simulink model "controlGPI_pos_6dof_sinMI"  (R2023b)
settings: Solver=ode45  StartTime=0.0  StopTime=tsim  FixedStep=tstep  MaxStep=tstep  RelTol=tstep/10
undefined symbols (not defined in the file): contr_robot_params, ddq, dq, ndof, NN_Bspline_params, NN_RBF_params, nn_select, Pc, q0, q_cero, q_eq, robot_params, t_qeq_init, t_tr_init, t_trtr, tau_L, tau_L_mags, tr_muestra, tr_ref, Wc, Zc
libraries: simulink x2
(part 1 of 2)
settings Model: Creator=HP  LastModifiedBy=HP

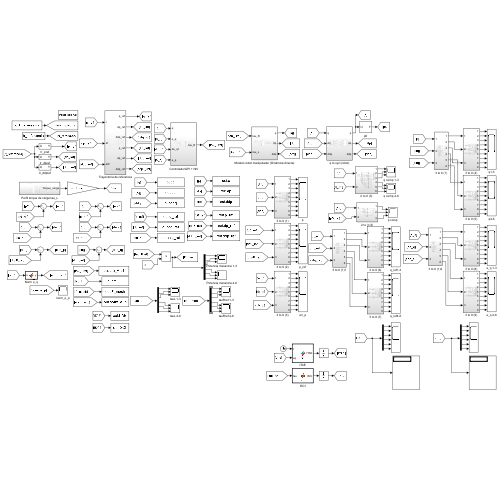
[thumbnail: Simulink's stored preview of the top-level diagram]
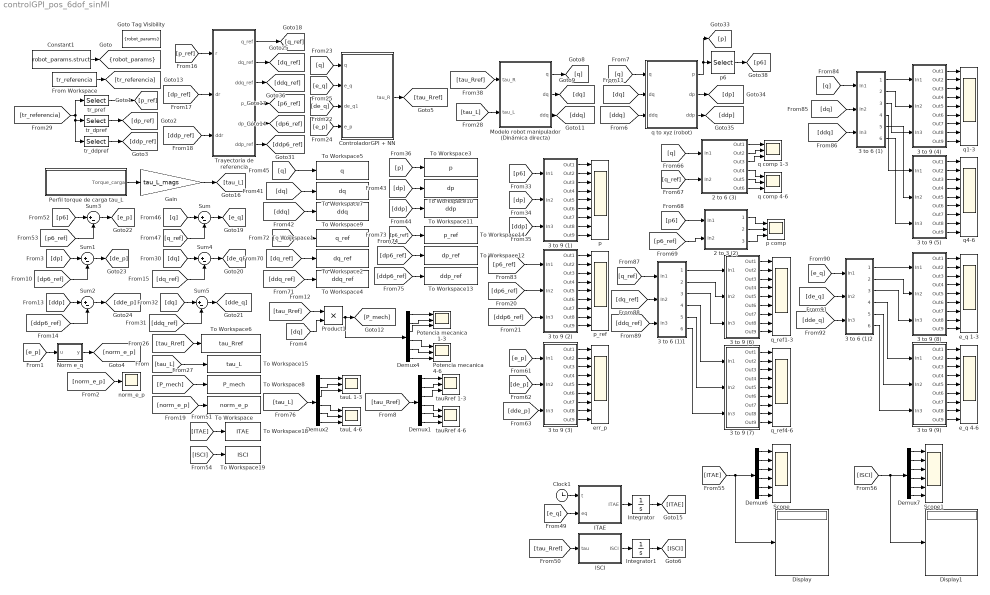
== system controlGPI_pos_6dof_sinMI ==
  2 to 3 (2) : Subsystem
  2 to 6 (3) : Subsystem
  3 to 6 (1) : Subsystem
  3 to 6 (1)1 : Subsystem
  3 to 6 (1)2 : Subsystem
  3 to 9 (1) : Subsystem
  3 to 9 (2) : Subsystem
  3 to 9 (3) : Subsystem
  3 to 9 (4) : Subsystem
  3 to 9 (5) : Subsystem
  3 to 9 (6) : Subsystem
  3 to 9 (7) : Subsystem
  3 to 9 (8) : Subsystem
  3 to 9 (9) : Subsystem
  Clock1 : Clock
  Constant1 : Constant  Value=robot_params.struct  OutDataTypeStr=Bus: robot_params_bus
  ControladorGPI + NN : Subsystem
  Demux{1..2,4,6..7} (5 alike) : Demux  Outputs=6
  Display : Display
  Display1 : Display
  From Workspace : FromWorkspace  VariableName=tr_referencia
  Gain : Gain  Gain=tau_L_mags
  Goto Tag Visibility : GotoTagVisibility  GotoTag=robot_params
  ISCI : MATLAB Function  TreatAsAtomicUnit=on
  ITAE : MATLAB Function  TreatAsAtomicUnit=on
  Integrator : Integrator
  Integrator1 : Integrator
  Modelo robot manipulador (Dinámica directa) : Subsystem
  Norm e_q : MATLAB Function  TreatAsAtomicUnit=on
  Perfil torque de carga tau_L : Subsystem
  Potencia mecanica 1-3 : Scope  NumInputPorts=3
  Potencia mecanica 4-6 : Scope  NumInputPorts=3
  Product1 : Product
  Scope : Scope  NumInputPorts=6
  Scope1 : Scope  NumInputPorts=6
  Sum{,1..5} (6 alike) : Sum  Inputs=|+-
  To Workspace : ToWorkspace  VariableName=norm_e_p  SaveFormat=Timeseries  SampleTime=-1
  To Workspace1 : ToWorkspace  VariableName=q_ref  SaveFormat=Timeseries  SampleTime=-1
  To Workspace10 : ToWorkspace  VariableName=dp  SaveFormat=Timeseries  SampleTime=-1
  To Workspace11 : ToWorkspace  VariableName=ddp  SaveFormat=Timeseries  SampleTime=-1
  To Workspace12 : ToWorkspace  VariableName=dp_ref  SaveFormat=Timeseries  SampleTime=-1
  To Workspace13 : ToWorkspace  VariableName=ddp_ref  SaveFormat=Timeseries  SampleTime=-1
  To Workspace14 : ToWorkspace  VariableName=p_ref  SaveFormat=Timeseries  SampleTime=-1
  To Workspace15 : ToWorkspace  VariableName=tau_L  SaveFormat=Timeseries  SampleTime=-1
  To Workspace18 : ToWorkspace  VariableName=ITAE  SampleTime=-1
      settings: MaxDataPoints=1
  To Workspace19 : ToWorkspace  VariableName=ISCI  SampleTime=-1
      settings: MaxDataPoints=1
  To Workspace2 : ToWorkspace  VariableName=dq_ref  SaveFormat=Timeseries  SampleTime=-1
  To Workspace3 : ToWorkspace  VariableName=p  SaveFormat=Timeseries  SampleTime=-1
  To Workspace4 : ToWorkspace  VariableName=ddq_ref  SaveFormat=Timeseries  SampleTime=-1
  To Workspace5 : ToWorkspace  VariableName=q  SaveFormat=Timeseries  SampleTime=-1
  To Workspace6 : ToWorkspace  VariableName=tau_Rref  SaveFormat=Timeseries  SampleTime=-1
  To Workspace7 : ToWorkspace  VariableName=dq  SaveFormat=Timeseries  SampleTime=-1
  To Workspace8 : ToWorkspace  VariableName=P_mech  SaveFormat=Timeseries  SampleTime=-1
  To Workspace9 : ToWorkspace  VariableName=ddq  SaveFormat=Timeseries  SampleTime=-1
  Trayectoria de referencia : Subsystem
  e_q 1-3 : Scope  NumInputPorts=9
  e_q 4-6 : Scope  NumInputPorts=9
  err_p : Scope  NumInputPorts=9
  norm_e_p : Scope
  p : Scope  NumInputPorts=9
  p comp : Scope  NumInputPorts=3
  p6 : Selector  NumberOfDimensions=2  InputPortWidth=3  IndexOptions=Index vector (dialog),Index vector (dialog)  Indices=[1:3],6  OutputSizes=1,1
  p_ref : Scope  NumInputPorts=9
  q comp 1-3 : Scope  NumInputPorts=3
  q comp 4-6 : Scope  NumInputPorts=3
  q to xyz (robot) : Subsystem
  q1-3 : Scope  NumInputPorts=9
  q4-6 : Scope  NumInputPorts=9
  q_ref1-3 : Scope  NumInputPorts=9
  q_ref4-6 : Scope  NumInputPorts=9
  tauL 1-3 : Scope  NumInputPorts=3
  tauL 4-6 : Scope  NumInputPorts=3
  tauRref 1-3 : Scope  NumInputPorts=3
  tauRref 4-6 : Scope  NumInputPorts=3
  tr_ddpref : Selector  NumberOfDimensions=2  InputPortWidth=3  IndexOptions=Index vector (dialog),Index vector (dialog)  Indices=[7:9],1  OutputSizes=1,1
  tr_dpref : Selector  NumberOfDimensions=2  InputPortWidth=3  IndexOptions=Index vector (dialog),Index vector (dialog)  Indices=[4:6],1  OutputSizes=1,1
  tr_pref : Selector  NumberOfDimensions=2  InputPortWidth=3  IndexOptions=Index vector (dialog),Index vector (dialog)  Indices=[1:3],1  OutputSizes=1,1
  tag scope: robot_params=scoped
  wires:
  [ddp] -> To Workspace11/1
  [P_mech] -> To Workspace8/1
  [dq] -> To Workspace7/1
  [q] -> To Workspace5/1
  [tau_Rref] -> To Workspace6/1
  [dp] -> To Workspace10/1
  [p] -> To Workspace3/1
  [ddq] -> To Workspace9/1
  [dq_ref] -> To Workspace2/1
  [ddq_ref] -> To Workspace4/1
  [q_ref] -> To Workspace1/1
  [p6_ref] -> To Workspace14/1
  [dp6_ref] -> To Workspace12/1
  [ddp6_ref] -> To Workspace13/1
  [tau_Rref] -> Modelo robot manipulador (Dinámica directa)/1(tau_R)
  [tau_L] -> Modelo robot manipulador (Dinámica directa)/2(tau_L)
  p6/1 -> [p6]
  q to xyz (robot)/1(p) -> p6/1, [p]
  [q] -> q to xyz (robot)/1(q)
  [dq] -> q to xyz (robot)/2(dq)
  [ddq] -> q to xyz (robot)/3(ddq)
  q to xyz (robot)/2(dp) -> [dp]
  q to xyz (robot)/3(ddp) -> [ddp]
  Modelo robot manipulador (Dinámica directa)/3(ddq) -> [ddq]
  Modelo robot manipulador (Dinámica directa)/2(dq) -> [dq]
  Modelo robot manipulador (Dinámica directa)/1(q) -> [q]
  2 to 6 (3)/6(Out6) -> q comp 4-6/3
  Demux4/2 -> Potencia mecanica 1-3/2
  2 to 6 (3)/5(Out5) -> q comp 4-6/2
  Demux1/4 -> tauRref 4-6/1
  2 to 6 (3)/3(Out3) -> q comp 1-3/3
  2 to 6 (3)/2(Out2) -> q comp 1-3/2
  3 to 9 (1)/4(Out4) -> p/4
  3 to 9 (2)/3(Out3) -> p_ref/3
  3 to 9 (3)/3(Out3) -> err_p/3
  3 to 9 (7)/9(Out9) -> q_ref4-6/9
  3 to 9 (4)/4(Out4) -> q1-3/4
  Demux2/5 -> tauL 4-6/2
  [tau_Rref] -> Demux1/1
  3 to 9 (1)/2(Out2) -> p/2
  [de_q] -> 3 to 6 (1)2/2(In2)
  Demux4/3 -> Potencia mecanica 1-3/3
  3 to 9 (3)/8(Out8) -> err_p/8
  2 to 3 (2)/3(3) -> p comp/3
  3 to 9 (5)/4(Out4) -> q4-6/4
  3 to 6 (1)/4(Out4) -> 3 to 9 (5)/1(In1)
  [dq] -> Product1/2
  3 to 6 (1)2/1(Out1) -> 3 to 9 (8)/1(In1)
  Demux2/3 -> tauL 1-3/3
  3 to 9 (6)/9(Out9) -> q_ref1-3/9
  3 to 9 (3)/4(Out4) -> err_p/4
  3 to 9 (7)/4(Out4) -> q_ref4-6/4
  3 to 9 (4)/1(Out1) -> q1-3/1
  3 to 9 (1)/9(Out9) -> p/9
  3 to 9 (2)/7(Out7) -> p_ref/7
  Product1/1 -> Demux4/1, [P_mech]
  Demux4/6 -> Potencia mecanica 4-6/3
  3 to 9 (1)/7(Out7) -> p/7
  3 to 9 (1)/6(Out6) -> p/6
  [dde_p] -> 3 to 9 (3)/3(In3)
  Demux4/4 -> Potencia mecanica 4-6/1
  3 to 9 (7)/1(Out1) -> q_ref4-6/1
  3 to 9 (4)/8(Out8) -> q1-3/8
  3 to 9 (4)/3(Out3) -> q1-3/3
  Demux2/1 -> tauL 1-3/1
  3 to 9 (2)/5(Out5) -> p_ref/5
  Demux1/1 -> tauRref 1-3/1
  3 to 9 (2)/9(Out9) -> p_ref/9
  3 to 6 (1)1/3(Out3) -> 3 to 9 (6)/3(In3)
  3 to 6 (1)/5(Out5) -> 3 to 9 (5)/2(In2)
  3 to 9 (5)/8(Out8) -> q4-6/8
  3 to 9 (4)/5(Out5) -> q1-3/5
  3 to 6 (1)1/1(Out1) -> 3 to 9 (6)/1(In1)
  3 to 9 (3)/2(Out2) -> err_p/2
  3 to 9 (8)/5(Out5) -> e_q 1-3/5
  3 to 9 (6)/1(Out1) -> q_ref1-3/1
  3 to 9 (2)/4(Out4) -> p_ref/4
  3 to 9 (5)/7(Out7) -> q4-6/7
  Demux2/4 -> tauL 4-6/1
  Demux2/2 -> tauL 1-3/2
  [ddp6_ref] -> 3 to 9 (2)/3(In3)
  Demux2/6 -> tauL 4-6/3
  3 to 6 (1)1/2(Out2) -> 3 to 9 (6)/2(In2)
  3 to 9 (7)/2(Out2) -> q_ref4-6/2
  3 to 9 (1)/1(Out1) -> p/1
  3 to 9 (3)/9(Out9) -> err_p/9
  3 to 9 (8)/1(Out1) -> e_q 1-3/1
  3 to 9 (3)/1(Out1) -> err_p/1
  3 to 9 (2)/6(Out6) -> p_ref/6
  Demux1/3 -> tauRref 1-3/3
  Demux1/5 -> tauRref 4-6/2
  3 to 9 (6)/4(Out4) -> q_ref1-3/4
  3 to 6 (1)1/5(Out5) -> 3 to 9 (7)/2(In2)
  Demux1/6 -> tauRref 4-6/3
  3 to 9 (8)/8(Out8) -> e_q 1-3/8
  3 to 9 (6)/3(Out3) -> q_ref1-3/3
  Demux1/2 -> tauRref 1-3/2
  3 to 6 (1)2/6(Out6) -> 3 to 9 (9)/3(In3)
  [tau_L] -> Demux2/1
  [dde_q] -> 3 to 6 (1)2/3(In3)
  3 to 9 (8)/2(Out2) -> e_q 1-3/2
  3 to 9 (8)/3(Out3) -> e_q 1-3/3
  3 to 9 (7)/3(Out3) -> q_ref4-6/3
  [de_p] -> 3 to 9 (3)/2(In2)
  [dp] -> 3 to 9 (1)/2(In2)
  3 to 9 (2)/8(Out8) -> p_ref/8
  3 to 6 (1)/1(Out1) -> 3 to 9 (4)/1(In1)
  3 to 9 (5)/3(Out3) -> q4-6/3
  [dq_ref] -> 3 to 6 (1)1/2(In2)
  3 to 9 (9)/8(Out8) -> e_q 4-6/8
  3 to 9 (6)/6(Out6) -> q_ref1-3/6
  3 to 9 (7)/8(Out8) -> q_ref4-6/8
  3 to 9 (8)/9(Out9) -> e_q 1-3/9
  [dp6_ref] -> 3 to 9 (2)/2(In2)
  3 to 9 (4)/6(Out6) -> q1-3/6
  3 to 9 (3)/6(Out6) -> err_p/6
  3 to 9 (6)/2(Out2) -> q_ref1-3/2
  3 to 9 (5)/6(Out6) -> q4-6/6
  3 to 6 (1)2/3(Out3) -> 3 to 9 (8)/3(In3)
  3 to 6 (1)1/4(Out4) -> 3 to 9 (7)/1(In1)
  3 to 9 (1)/8(Out8) -> p/8
  [tau_Rref] -> Product1/1
  3 to 9 (3)/7(Out7) -> err_p/7
  [q] -> 3 to 6 (1)/1(In1)
  2 to 3 (2)/1(1) -> p comp/1
  [ddq_ref] -> 3 to 6 (1)1/3(In3)
  3 to 9 (2)/2(Out2) -> p_ref/2
  3 to 9 (8)/4(Out4) -> e_q 1-3/4
  [dq] -> 3 to 6 (1)/2(In2)
  3 to 6 (1)2/2(Out2) -> 3 to 9 (8)/2(In2)
  3 to 9 (4)/7(Out7) -> q1-3/7
  [p6] -> 3 to 9 (1)/1(In1)
  3 to 6 (1)/6(Out6) -> 3 to 9 (5)/3(In3)
  3 to 9 (9)/5(Out5) -> e_q 4-6/5
  Demux4/5 -> Potencia mecanica 4-6/2
  3 to 9 (9)/4(Out4) -> e_q 4-6/4
  3 to 6 (1)2/4(Out4) -> 3 to 9 (9)/1(In1)
  3 to 9 (8)/6(Out6) -> e_q 1-3/6
  2 to 6 (3)/1(Out1) -> q comp 1-3/1
  [p6_ref] -> 3 to 9 (2)/1(In1)
  [e_p] -> 3 to 9 (3)/1(In1)
  2 to 6 (3)/4(Out4) -> q comp 4-6/1
  3 to 9 (1)/3(Out3) -> p/3
  3 to 6 (1)2/5(Out5) -> 3 to 9 (9)/2(In2)
  [p6] -> 2 to 3 (2)/1(In1)
  3 to 9 (4)/2(Out2) -> q1-3/2
  3 to 9 (9)/6(Out6) -> e_q 4-6/6
  [q] -> 2 to 6 (3)/1(In1)
  3 to 6 (1)/2(Out2) -> 3 to 9 (4)/2(In2)
  3 to 9 (3)/5(Out5) -> err_p/5
  3 to 9 (8)/7(Out7) -> e_q 1-3/7
  3 to 9 (5)/5(Out5) -> q4-6/5
  3 to 6 (1)1/6(Out6) -> 3 to 9 (7)/3(In3)
  3 to 9 (1)/5(Out5) -> p/5
  3 to 9 (2)/1(Out1) -> p_ref/1
  3 to 9 (7)/5(Out5) -> q_ref4-6/5
  3 to 9 (5)/9(Out9) -> q4-6/9
  3 to 9 (7)/6(Out6) -> q_ref4-6/6
  3 to 6 (1)/3(Out3) -> 3 to 9 (4)/3(In3)
  [q_ref] -> 2 to 6 (3)/2(In2)
  3 to 9 (9)/7(Out7) -> e_q 4-6/7
  2 to 3 (2)/2(2) -> p comp/2
  3 to 9 (7)/7(Out7) -> q_ref4-6/7
  3 to 9 (5)/1(Out1) -> q4-6/1
  3 to 9 (9)/3(Out3) -> e_q 4-6/3
  3 to 9 (4)/9(Out9) -> q1-3/9
  3 to 9 (6)/5(Out5) -> q_ref1-3/5
  Demux4/1 -> Potencia mecanica 1-3/1
  3 to 9 (6)/8(Out8) -> q_ref1-3/8
  3 to 9 (9)/2(Out2) -> e_q 4-6/2
  [ddp] -> 3 to 9 (1)/3(In3)
  [p6_ref] -> 2 to 3 (2)/2(In2)
  [e_q] -> 3 to 6 (1)2/1(In1)
  3 to 9 (9)/9(Out9) -> e_q 4-6/9
  3 to 9 (9)/1(Out1) -> e_q 4-6/1
  [q_ref] -> 3 to 6 (1)1/1(In1)
  3 to 9 (6)/7(Out7) -> q_ref1-3/7
  [ddq] -> 3 to 6 (1)/3(In3)
  3 to 9 (5)/2(Out2) -> q4-6/2
  tr_pref/1 -> [p_ref]
  tr_ddpref/1 -> [ddp_ref]
  [tr_referencia] -> tr_dpref/1, tr_ddpref/1, tr_pref/1
  Constant1/1 -> [robot_params]
  tr_dpref/1 -> [dp_ref]
  From Workspace/1 -> [tr_referencia]
  Trayectoria de referencia/4(p_ref) -> [p6_ref]
  Trayectoria de referencia/5(dp_ref) -> [dp6_ref]
  Trayectoria de referencia/3(ddq_ref) -> [ddq_ref]
  Trayectoria de referencia/2(dq_ref) -> [dq_ref]
  [p_ref] -> Trayectoria de referencia/1(r)
  [ddp_ref] -> Trayectoria de referencia/3(ddr)
  Trayectoria de referencia/6(ddp_ref) -> [ddp6_ref]
  Trayectoria de referencia/1(q_ref) -> [q_ref]
  [dp_ref] -> Trayectoria de referencia/2(dr)
  Sum1/1 -> [de_p]
  [norm_e_p] -> norm_e_p/1
  Sum2/1 -> [dde_p]
  Norm e_q/1(y) -> [norm_e_p]
  [p6] -> Sum3/1
  [q_ref] -> Sum/2
  Sum3/1 -> [e_p]
  Sum/1 -> [e_q]
  [e_p] -> Norm e_q/1(u)
  [q] -> Sum/1
  [p6_ref] -> Sum3/2
  [norm_e_p] -> To Workspace/1
  [e_q] -> ControladorGPI + NN/2(e_q)
  ControladorGPI + NN/1(tau_R) -> [tau_Rref]
  [de_q] -> ControladorGPI + NN/3(de_q1)
  [q] -> ControladorGPI + NN/1(q)
  [e_p] -> ControladorGPI + NN/4(e_p)
  [dp] -> Sum1/1
  [dp6_ref] -> Sum1/2
  [ddp] -> Sum2/1
  [ddp6_ref] -> Sum2/2
  [dq_ref] -> Sum4/2
  [dq] -> Sum4/1
  Sum4/1 -> [de_q]
  [ddq_ref] -> Sum5/2
  [dq] -> Sum5/1
  Sum5/1 -> [dde_q]
  Perfil torque de carga tau_L/1(Torque_carga) -> Gain/1
  Gain/1 -> [tau_L]
  [tau_L] -> To Workspace15/1
  Demux6/6 -> Scope/6
  Demux7/6 -> Scope1/6
  Demux7/5 -> Scope1/5
  ITAE/1(ITAE) -> Integrator/1
  [tau_Rref] -> ISCI/1(tau)
  Integrator/1 -> [ITAE]
  Integrator1/1 -> [ISCI]
  Demux6/5 -> Scope/5
  ISCI/1(ISCI) -> Integrator1/1
  [e_q] -> ITAE/2(eq)
  Clock1/1 -> ITAE/1(t)
  [ITAE] -> Display/1, Demux6/1
  [ISCI] -> Display1/1, Demux7/1
  Demux6/1 -> Scope/1
  Demux6/2 -> Scope/2
  Demux6/3 -> Scope/3
  Demux6/4 -> Scope/4
  Demux7/1 -> Scope1/1
  Demux7/2 -> Scope1/2
  Demux7/3 -> Scope1/3
  Demux7/4 -> Scope1/4
  [ITAE] -> To Workspace18/1
  [ISCI] -> To Workspace19/1

== system controlGPI_pos_6dof_sinMI/2 to 3 (2) ==
  In1 : Inport
  In2 : Inport  Port=2
  Demux3 : Demux  Outputs=3
  Demux4 : Demux  Outputs=3
  Mux10 : Mux  Inputs=2
  Mux8 : Mux  Inputs=2
  Mux9 : Mux  Inputs=2
  1 : Outport
  2 : Outport  Port=2
  3 : Outport  Port=3
  wires:
  Demux4/3 -> Mux10/2
  Demux3/1 -> Mux8/1
  Demux3/2 -> Mux9/1
  Mux9/1 -> 2/1
  Demux4/2 -> Mux9/2
  Demux4/1 -> Mux8/2
  Demux3/3 -> Mux10/1
  Mux8/1 -> 1/1
  Mux10/1 -> 3/1
  In1/1 -> Demux3/1
  In2/1 -> Demux4/1

== system controlGPI_pos_6dof_sinMI/2 to 6 (3) ==
  In1 : Inport
  In2 : Inport  Port=2
  Demux4 : Demux  Outputs=6
  Demux6 : Demux  Outputs=6
  Mux{,1..5} (6 alike) : Mux  Inputs=2
  Out1 : Outport
  Out2 : Outport  Port=2
  Out3 : Outport  Port=3
  Out4 : Outport  Port=4
  Out5 : Outport  Port=5
  Out6 : Outport  Port=6
  wires:
  In2/1 -> Demux6/1
  Demux4/3 -> Mux2/1
  Demux4/5 -> Mux4/1
  Demux4/6 -> Mux5/1
  Demux6/5 -> Mux4/2
  Demux4/1 -> Mux/1
  Demux6/6 -> Mux5/2
  In1/1 -> Demux4/1
  Demux4/4 -> Mux3/1
  Demux6/2 -> Mux1/2
  Demux6/4 -> Mux3/2
  Demux6/1 -> Mux/2
  Demux4/2 -> Mux1/1
  Demux6/3 -> Mux2/2
  Mux/1 -> Out1/1
  Mux1/1 -> Out2/1
  Mux2/1 -> Out3/1
  Mux3/1 -> Out4/1
  Mux4/1 -> Out5/1
  Mux5/1 -> Out6/1

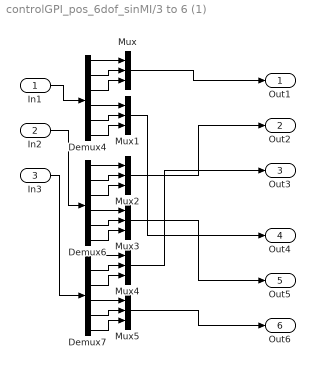
== system controlGPI_pos_6dof_sinMI/3 to 6 (1) ==
  In1 : Inport
  In2 : Inport  Port=2
  In3 : Inport  Port=3
  Demux4 : Demux  Outputs=6
  Demux6 : Demux  Outputs=6
  Demux7 : Demux  Outputs=6
  Mux{,1..5} (6 alike) : Mux  Inputs=3
  Out1 : Outport
  Out2 : Outport  Port=2
  Out3 : Outport  Port=3
  Out4 : Outport  Port=4
  Out5 : Outport  Port=5
  Out6 : Outport  Port=6
  wires:
  Demux6/1 -> Mux2/1
  Demux6/3 -> Mux2/3
  Demux4/2 -> Mux/2
  Demux6/6 -> Mux3/3
  Demux6/2 -> Mux2/2
  Demux6/5 -> Mux3/2
  Mux/1 -> Out1/1
  In1/1 -> Demux4/1
  Demux6/4 -> Mux3/1
  Demux4/1 -> Mux/1
  Demux4/6 -> Mux1/3
  Demux4/4 -> Mux1/1
  Demux7/5 -> Mux5/2
  Demux4/3 -> Mux/3
  Demux4/5 -> Mux1/2
  Demux7/3 -> Mux4/3
  Demux7/1 -> Mux4/1
  Demux7/2 -> Mux4/2
  In3/1 -> Demux7/1
  Mux2/1 -> Out2/1
  Demux7/4 -> Mux5/1
  Demux7/6 -> Mux5/3
  In2/1 -> Demux6/1
  Mux5/1 -> Out6/1
  Mux1/1 -> Out4/1
  Mux4/1 -> Out3/1
  Mux3/1 -> Out5/1

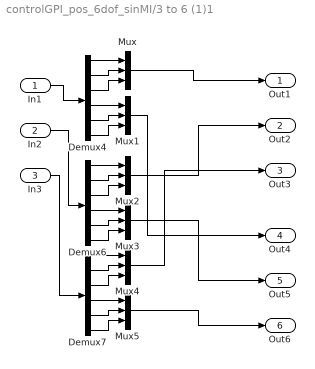
== system controlGPI_pos_6dof_sinMI/3 to 6 (1)1 ==
  In1 : Inport
  In2 : Inport  Port=2
  In3 : Inport  Port=3
  Demux4 : Demux  Outputs=6
  Demux6 : Demux  Outputs=6
  Demux7 : Demux  Outputs=6
  Mux{,1..5} (6 alike) : Mux  Inputs=3
  Out1 : Outport
  Out2 : Outport  Port=2
  Out3 : Outport  Port=3
  Out4 : Outport  Port=4
  Out5 : Outport  Port=5
  Out6 : Outport  Port=6
  wires:
  Demux6/1 -> Mux2/1
  Demux6/3 -> Mux2/3
  Demux4/2 -> Mux/2
  Demux6/6 -> Mux3/3
  Demux6/2 -> Mux2/2
  Demux6/5 -> Mux3/2
  Mux/1 -> Out1/1
  In1/1 -> Demux4/1
  Demux6/4 -> Mux3/1
  Demux4/1 -> Mux/1
  Demux4/6 -> Mux1/3
  Demux4/4 -> Mux1/1
  Demux7/5 -> Mux5/2
  Demux4/3 -> Mux/3
  Demux4/5 -> Mux1/2
  Demux7/3 -> Mux4/3
  Demux7/1 -> Mux4/1
  Demux7/2 -> Mux4/2
  In3/1 -> Demux7/1
  Mux2/1 -> Out2/1
  Demux7/4 -> Mux5/1
  Demux7/6 -> Mux5/3
  In2/1 -> Demux6/1
  Mux5/1 -> Out6/1
  Mux1/1 -> Out4/1
  Mux4/1 -> Out3/1
  Mux3/1 -> Out5/1

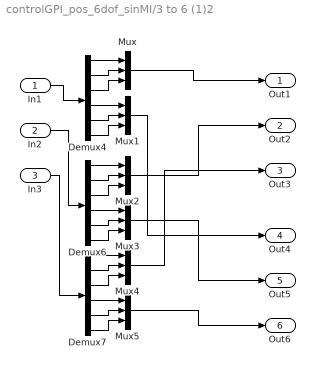
== system controlGPI_pos_6dof_sinMI/3 to 6 (1)2 ==
  In1 : Inport
  In2 : Inport  Port=2
  In3 : Inport  Port=3
  Demux4 : Demux  Outputs=6
  Demux6 : Demux  Outputs=6
  Demux7 : Demux  Outputs=6
  Mux{,1..5} (6 alike) : Mux  Inputs=3
  Out1 : Outport
  Out2 : Outport  Port=2
  Out3 : Outport  Port=3
  Out4 : Outport  Port=4
  Out5 : Outport  Port=5
  Out6 : Outport  Port=6
  wires:
  Demux6/1 -> Mux2/1
  Demux6/3 -> Mux2/3
  Demux4/2 -> Mux/2
  Demux6/6 -> Mux3/3
  Demux6/2 -> Mux2/2
  Demux6/5 -> Mux3/2
  Mux/1 -> Out1/1
  In1/1 -> Demux4/1
  Demux6/4 -> Mux3/1
  Demux4/1 -> Mux/1
  Demux4/6 -> Mux1/3
  Demux4/4 -> Mux1/1
  Demux7/5 -> Mux5/2
  Demux4/3 -> Mux/3
  Demux4/5 -> Mux1/2
  Demux7/3 -> Mux4/3
  Demux7/1 -> Mux4/1
  Demux7/2 -> Mux4/2
  In3/1 -> Demux7/1
  Mux2/1 -> Out2/1
  Demux7/4 -> Mux5/1
  Demux7/6 -> Mux5/3
  In2/1 -> Demux6/1
  Mux5/1 -> Out6/1
  Mux1/1 -> Out4/1
  Mux4/1 -> Out3/1
  Mux3/1 -> Out5/1

== system controlGPI_pos_6dof_sinMI/3 to 9 (1) ==
  In1 : Inport
  In2 : Inport  Port=2
  In3 : Inport  Port=3
  Demux2 : Demux  Outputs=3
  Demux3 : Demux  Outputs=3
  Demux4 : Demux  Outputs=3
  Out1 : Outport
  Out2 : Outport  Port=2
  Out3 : Outport  Port=3
  Out4 : Outport  Port=4
  Out5 : Outport  Port=5
  Out6 : Outport  Port=6
  Out7 : Outport  Port=7
  Out8 : Outport  Port=8
  Out9 : Outport  Port=9
  wires:
  In3/1 -> Demux4/1
  Demux4/1 -> Out3/1
  Demux2/1 -> Out1/1
  Demux3/3 -> Out8/1
  Demux3/2 -> Out5/1
  Demux3/1 -> Out2/1
  In1/1 -> Demux2/1
  Demux2/3 -> Out7/1
  Demux4/3 -> Out9/1
  Demux4/2 -> Out6/1
  Demux2/2 -> Out4/1
  In2/1 -> Demux3/1

== system controlGPI_pos_6dof_sinMI/3 to 9 (2) ==
  In1 : Inport
  In2 : Inport  Port=2
  In3 : Inport  Port=3
  Demux2 : Demux  Outputs=3
  Demux3 : Demux  Outputs=3
  Demux4 : Demux  Outputs=3
  Out1 : Outport
  Out2 : Outport  Port=2
  Out3 : Outport  Port=3
  Out4 : Outport  Port=4
  Out5 : Outport  Port=5
  Out6 : Outport  Port=6
  Out7 : Outport  Port=7
  Out8 : Outport  Port=8
  Out9 : Outport  Port=9
  wires:
  In3/1 -> Demux4/1
  Demux4/1 -> Out3/1
  Demux2/1 -> Out1/1
  Demux3/3 -> Out8/1
  Demux3/2 -> Out5/1
  Demux3/1 -> Out2/1
  In1/1 -> Demux2/1
  Demux2/3 -> Out7/1
  Demux4/3 -> Out9/1
  Demux4/2 -> Out6/1
  Demux2/2 -> Out4/1
  In2/1 -> Demux3/1

== system controlGPI_pos_6dof_sinMI/3 to 9 (3) ==
  In1 : Inport
  In2 : Inport  Port=2
  In3 : Inport  Port=3
  Demux2 : Demux  Outputs=3
  Demux3 : Demux  Outputs=3
  Demux4 : Demux  Outputs=3
  Out1 : Outport
  Out2 : Outport  Port=2
  Out3 : Outport  Port=3
  Out4 : Outport  Port=4
  Out5 : Outport  Port=5
  Out6 : Outport  Port=6
  Out7 : Outport  Port=7
  Out8 : Outport  Port=8
  Out9 : Outport  Port=9
  wires:
  In3/1 -> Demux4/1
  Demux4/1 -> Out3/1
  Demux2/1 -> Out1/1
  Demux3/3 -> Out8/1
  Demux3/2 -> Out5/1
  Demux3/1 -> Out2/1
  In1/1 -> Demux2/1
  Demux2/3 -> Out7/1
  Demux4/3 -> Out9/1
  Demux4/2 -> Out6/1
  Demux2/2 -> Out4/1
  In2/1 -> Demux3/1

== system controlGPI_pos_6dof_sinMI/3 to 9 (4) ==
  In1 : Inport
  In2 : Inport  Port=2
  In3 : Inport  Port=3
  Demux2 : Demux  Outputs=3
  Demux3 : Demux  Outputs=3
  Demux4 : Demux  Outputs=3
  Out1 : Outport
  Out2 : Outport  Port=2
  Out3 : Outport  Port=3
  Out4 : Outport  Port=4
  Out5 : Outport  Port=5
  Out6 : Outport  Port=6
  Out7 : Outport  Port=7
  Out8 : Outport  Port=8
  Out9 : Outport  Port=9
  wires:
  In3/1 -> Demux4/1
  Demux4/1 -> Out3/1
  Demux2/1 -> Out1/1
  Demux3/3 -> Out8/1
  Demux3/2 -> Out5/1
  Demux3/1 -> Out2/1
  In1/1 -> Demux2/1
  Demux2/3 -> Out7/1
  Demux4/3 -> Out9/1
  Demux4/2 -> Out6/1
  Demux2/2 -> Out4/1
  In2/1 -> Demux3/1

== system controlGPI_pos_6dof_sinMI/3 to 9 (5) ==
  In1 : Inport
  In2 : Inport  Port=2
  In3 : Inport  Port=3
  Demux2 : Demux  Outputs=3
  Demux3 : Demux  Outputs=3
  Demux4 : Demux  Outputs=3
  Out1 : Outport
  Out2 : Outport  Port=2
  Out3 : Outport  Port=3
  Out4 : Outport  Port=4
  Out5 : Outport  Port=5
  Out6 : Outport  Port=6
  Out7 : Outport  Port=7
  Out8 : Outport  Port=8
  Out9 : Outport  Port=9
  wires:
  In3/1 -> Demux4/1
  Demux4/1 -> Out3/1
  Demux2/1 -> Out1/1
  Demux3/3 -> Out8/1
  Demux3/2 -> Out5/1
  Demux3/1 -> Out2/1
  In1/1 -> Demux2/1
  Demux2/3 -> Out7/1
  Demux4/3 -> Out9/1
  Demux4/2 -> Out6/1
  Demux2/2 -> Out4/1
  In2/1 -> Demux3/1

== system controlGPI_pos_6dof_sinMI/3 to 9 (6) ==
  In1 : Inport
  In2 : Inport  Port=2
  In3 : Inport  Port=3
  Demux2 : Demux  Outputs=3
  Demux3 : Demux  Outputs=3
  Demux4 : Demux  Outputs=3
  Out1 : Outport
  Out2 : Outport  Port=2
  Out3 : Outport  Port=3
  Out4 : Outport  Port=4
  Out5 : Outport  Port=5
  Out6 : Outport  Port=6
  Out7 : Outport  Port=7
  Out8 : Outport  Port=8
  Out9 : Outport  Port=9
  wires:
  In3/1 -> Demux4/1
  Demux4/1 -> Out3/1
  Demux2/1 -> Out1/1
  Demux3/3 -> Out8/1
  Demux3/2 -> Out5/1
  Demux3/1 -> Out2/1
  In1/1 -> Demux2/1
  Demux2/3 -> Out7/1
  Demux4/3 -> Out9/1
  Demux4/2 -> Out6/1
  Demux2/2 -> Out4/1
  In2/1 -> Demux3/1

== system controlGPI_pos_6dof_sinMI/3 to 9 (7) ==
  In1 : Inport
  In2 : Inport  Port=2
  In3 : Inport  Port=3
  Demux2 : Demux  Outputs=3
  Demux3 : Demux  Outputs=3
  Demux4 : Demux  Outputs=3
  Out1 : Outport
  Out2 : Outport  Port=2
  Out3 : Outport  Port=3
  Out4 : Outport  Port=4
  Out5 : Outport  Port=5
  Out6 : Outport  Port=6
  Out7 : Outport  Port=7
  Out8 : Outport  Port=8
  Out9 : Outport  Port=9
  wires:
  In3/1 -> Demux4/1
  Demux4/1 -> Out3/1
  Demux2/1 -> Out1/1
  Demux3/3 -> Out8/1
  Demux3/2 -> Out5/1
  Demux3/1 -> Out2/1
  In1/1 -> Demux2/1
  Demux2/3 -> Out7/1
  Demux4/3 -> Out9/1
  Demux4/2 -> Out6/1
  Demux2/2 -> Out4/1
  In2/1 -> Demux3/1

== system controlGPI_pos_6dof_sinMI/3 to 9 (8) ==
  In1 : Inport
  In2 : Inport  Port=2
  In3 : Inport  Port=3
  Demux2 : Demux  Outputs=3
  Demux3 : Demux  Outputs=3
  Demux4 : Demux  Outputs=3
  Out1 : Outport
  Out2 : Outport  Port=2
  Out3 : Outport  Port=3
  Out4 : Outport  Port=4
  Out5 : Outport  Port=5
  Out6 : Outport  Port=6
  Out7 : Outport  Port=7
  Out8 : Outport  Port=8
  Out9 : Outport  Port=9
  wires:
  In3/1 -> Demux4/1
  Demux4/1 -> Out3/1
  Demux2/1 -> Out1/1
  Demux3/3 -> Out8/1
  Demux3/2 -> Out5/1
  Demux3/1 -> Out2/1
  In1/1 -> Demux2/1
  Demux2/3 -> Out7/1
  Demux4/3 -> Out9/1
  Demux4/2 -> Out6/1
  Demux2/2 -> Out4/1
  In2/1 -> Demux3/1

== system controlGPI_pos_6dof_sinMI/3 to 9 (9) ==
  In1 : Inport
  In2 : Inport  Port=2
  In3 : Inport  Port=3
  Demux2 : Demux  Outputs=3
  Demux3 : Demux  Outputs=3
  Demux4 : Demux  Outputs=3
  Out1 : Outport
  Out2 : Outport  Port=2
  Out3 : Outport  Port=3
  Out4 : Outport  Port=4
  Out5 : Outport  Port=5
  Out6 : Outport  Port=6
  Out7 : Outport  Port=7
  Out8 : Outport  Port=8
  Out9 : Outport  Port=9
  wires:
  In3/1 -> Demux4/1
  Demux4/1 -> Out3/1
  Demux2/1 -> Out1/1
  Demux3/3 -> Out8/1
  Demux3/2 -> Out5/1
  Demux3/1 -> Out2/1
  In1/1 -> Demux2/1
  Demux2/3 -> Out7/1
  Demux4/3 -> Out9/1
  Demux4/2 -> Out6/1
  Demux2/2 -> Out4/1
  In2/1 -> Demux3/1

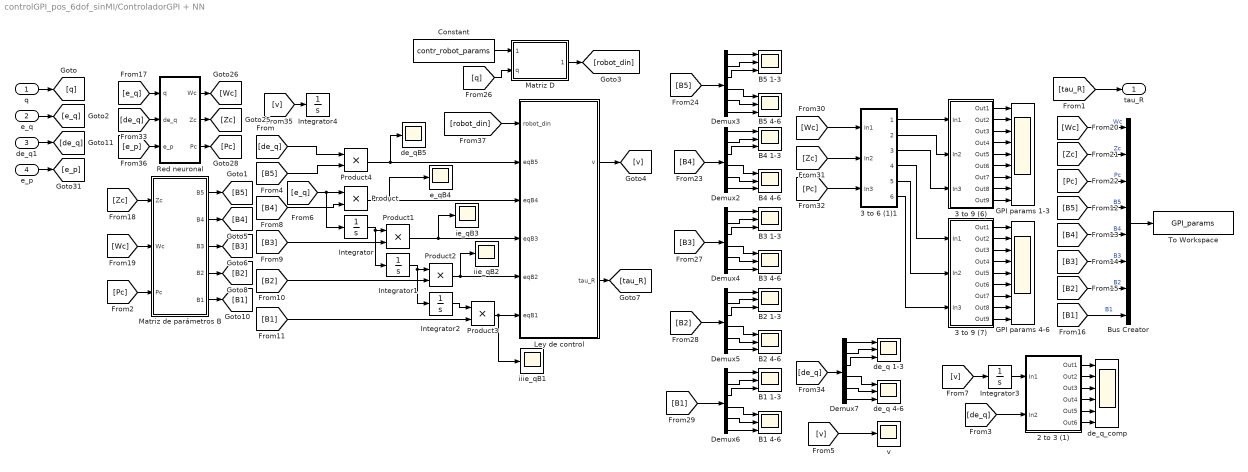
== system controlGPI_pos_6dof_sinMI/ControladorGPI + NN ==
  q : Inport
  e_q : Inport  Port=2
  de_q1 : Inport  Port=3
  e_p : Inport  Port=4
  2 to 3 (1) : Subsystem
  3 to 6 (1)1 : Subsystem
  3 to 9 (6) : Subsystem
  3 to 9 (7) : Subsystem
  B1 1-3 : Scope  NumInputPorts=3
  B1 4-6 : Scope  NumInputPorts=3
  B2 1-3 : Scope  NumInputPorts=3
  B2 4-6 : Scope  NumInputPorts=3
  B3 1-3 : Scope  NumInputPorts=3
  B3 4-6 : Scope  NumInputPorts=3
  B4 1-3 : Scope  NumInputPorts=3
  B4 4-6 : Scope  NumInputPorts=3
  B5 1-3 : Scope  NumInputPorts=3
  B5 4-6 : Scope  NumInputPorts=3
  Bus Creator : BusCreator  Inputs=8
  Constant : Constant  Value=contr_robot_params  OutDataTypeStr=Bus: robot_params_bus
  Demux{2..7} (6 alike) : Demux  Outputs=6
  GPI params 1-3 : Scope  NumInputPorts=9
  GPI params 4-6 : Scope  NumInputPorts=9
  Integrator{,1..4} (5 alike) : Integrator
  Ley de control : MATLAB Function  TreatAsAtomicUnit=on
  Matriz D : MATLAB Function  TreatAsAtomicUnit=on
  Matriz de parámetros B : MATLAB Function  TreatAsAtomicUnit=on
  Product{,1..4} (5 alike) : Product
  Red neuronal : Subsystem
  To Workspace : ToWorkspace  VariableName=GPI_params  SaveFormat=Timeseries  SampleTime=-1
  de_q 1-3 : Scope  NumInputPorts=3
  de_q 4-6 : Scope  NumInputPorts=3
  de_qB5 : Scope
  de_q_comp : Scope  NumInputPorts=6
  e_qB4 : Scope
  ie_qB3 : Scope
  iie_qB2 : Scope
  iiie_qB1 : Scope
  v : Scope
  tau_R : Outport
  wires:
  Ley de control/2(tau_R) -> [tau_R]
  [tau_R] -> tau_R/1
  e_q/1 -> [e_q]
  [e_q] -> Integrator/1, Product/1
  Integrator/1 -> Integrator1/1, Product1/1
  Integrator1/1 -> Integrator2/1, Product2/1
  Integrator2/1 -> Product3/1
  Product3/1 -> iiie_qB1/1, Ley de control/6(eqB1)
  Product2/1 -> iie_qB2/1, Ley de control/5(eqB2)
  Product1/1 -> ie_qB3/1, Ley de control/4(eqB3)
  Product/1 -> e_qB4/1, Ley de control/3(eqB4)
  Ley de control/1(v) -> [v]
  Product4/1 -> de_qB5/1, Ley de control/2(eqB5)
  [Zc] -> Matriz de parámetros B/1(Zc)
  [Wc] -> Matriz de parámetros B/2(Wc)
  [Pc] -> Matriz de parámetros B/3(Pc)
  Matriz de parámetros B/1(B5) -> [B5]
  Matriz de parámetros B/2(B4) -> [B4]
  Matriz de parámetros B/3(B3) -> [B3]
  Matriz de parámetros B/4(B2) -> [B2]
  Matriz de parámetros B/5(B1) -> [B1]
  [B5] -> Product4/2
  [B4] -> Product/2
  [B3] -> Product1/2
  [B2] -> Product2/2
  [B1] -> Product3/2
  Bus Creator/1 -> To Workspace/1
  [Wc] -> Bus Creator/1  "Wc"
  [Zc] -> Bus Creator/2  "Zc"
  [Pc] -> Bus Creator/3  "Pc"
  [B5] -> Bus Creator/4  "B5"
  [B4] -> Bus Creator/5  "B4"
  [B3] -> Bus Creator/6  "B3"
  [B2] -> Bus Creator/7  "B2"
  [B1] -> Bus Creator/8  "B1"
  Red neuronal/2(Zc) -> [Zc]
  Red neuronal/1(Wc) -> [Wc]
  Red neuronal/3(Pc) -> [Pc]
  [de_q] -> Red neuronal/2(de_q)
  [e_q] -> Red neuronal/1(q)
  de_q1/1 -> [de_q]
  e_p/1 -> [e_p]
  [e_p] -> Red neuronal/3(e_p)
  [q] -> Matriz D/2(q)
  q/1 -> [q]
  [v] -> Integrator3/1
  Integrator3/1 -> 2 to 3 (1)/1(In1)
  [de_q] -> 2 to 3 (1)/2(In2)
  [v] -> v/1
  [v] -> Integrator4/1
  3 to 6 (1)1/3(Out3) -> 3 to 9 (6)/3(In3)
  3 to 9 (6)/8(Out8) -> GPI params 1-3/8
  3 to 9 (6)/2(Out2) -> GPI params 1-3/2
  [Pc] -> 3 to 6 (1)1/3(In3)
  3 to 9 (6)/6(Out6) -> GPI params 1-3/6
  3 to 6 (1)1/4(Out4) -> 3 to 9 (7)/1(In1)
  3 to 9 (6)/7(Out7) -> GPI params 1-3/7
  3 to 6 (1)1/2(Out2) -> 3 to 9 (6)/2(In2)
  3 to 9 (6)/1(Out1) -> GPI params 1-3/1
  3 to 6 (1)1/6(Out6) -> 3 to 9 (7)/3(In3)
  3 to 9 (7)/4(Out4) -> GPI params 4-6/4
  3 to 9 (6)/9(Out9) -> GPI params 1-3/9
  [Wc] -> 3 to 6 (1)1/1(In1)
  3 to 9 (6)/4(Out4) -> GPI params 1-3/4
  3 to 6 (1)1/1(Out1) -> 3 to 9 (6)/1(In1)
  3 to 6 (1)1/5(Out5) -> 3 to 9 (7)/2(In2)
  3 to 9 (6)/3(Out3) -> GPI params 1-3/3
  3 to 9 (7)/1(Out1) -> GPI params 4-6/1
  3 to 9 (7)/3(Out3) -> GPI params 4-6/3
  3 to 9 (7)/2(Out2) -> GPI params 4-6/2
  3 to 9 (6)/5(Out5) -> GPI params 1-3/5
  [Zc] -> 3 to 6 (1)1/2(In2)
  3 to 9 (7)/5(Out5) -> GPI params 4-6/5
  3 to 9 (7)/6(Out6) -> GPI params 4-6/6
  3 to 9 (7)/7(Out7) -> GPI params 4-6/7
  3 to 9 (7)/8(Out8) -> GPI params 4-6/8
  3 to 9 (7)/9(Out9) -> GPI params 4-6/9
  Demux3/1 -> B5 1-3/1
  Demux6/5 -> B1 4-6/2
  Demux2/6 -> B4 4-6/3
  Demux5/3 -> B2 1-3/3
  [B2] -> Demux5/1
  Demux5/5 -> B2 4-6/2
  Demux6/6 -> B1 4-6/3
  Demux5/4 -> B2 4-6/1
  Demux3/6 -> B5 4-6/3
  [B1] -> Demux6/1
  Demux4/1 -> B3 1-3/1
  Demux4/3 -> B3 1-3/3
  [B3] -> Demux4/1
  Demux6/1 -> B1 1-3/1
  Demux6/3 -> B1 1-3/3
  [B4] -> Demux2/1
  [B5] -> Demux3/1
  Demux4/6 -> B3 4-6/3
  Demux5/2 -> B2 1-3/2
  Demux6/2 -> B1 1-3/2
  Demux6/4 -> B1 4-6/1
  Demux2/4 -> B4 4-6/1
  Demux4/4 -> B3 4-6/1
  Demux4/5 -> B3 4-6/2
  Demux2/1 -> B4 1-3/1
  Demux3/2 -> B5 1-3/2
  Demux2/5 -> B4 4-6/2
  Demux5/6 -> B2 4-6/3
  Demux2/2 -> B4 1-3/2
  Demux4/2 -> B3 1-3/2
  Demux3/4 -> B5 4-6/1
  Demux3/3 -> B5 1-3/3
  Demux2/3 -> B4 1-3/3
  Demux3/5 -> B5 4-6/2
  Demux5/1 -> B2 1-3/1
  Demux7/5 -> de_q 4-6/2
  Demux7/2 -> de_q 1-3/2
  Demux7/4 -> de_q 4-6/1
  Demux7/6 -> de_q 4-6/3
  Demux7/3 -> de_q 1-3/3
  [de_q] -> Demux7/1
  Demux7/1 -> de_q 1-3/1
  [de_q] -> Product4/1
  Constant/1 -> Matriz D/1(robot_params)
  Matriz D/1(robot_din) -> [robot_din]
  [robot_din] -> Ley de control/1(robot_din)
  2 to 3 (1)/1(Out1) -> de_q_comp/1
  2 to 3 (1)/2(Out2) -> de_q_comp/2
  2 to 3 (1)/3(Out3) -> de_q_comp/3
  2 to 3 (1)/4(Out4) -> de_q_comp/4
  2 to 3 (1)/5(Out5) -> de_q_comp/5
  2 to 3 (1)/6(Out6) -> de_q_comp/6

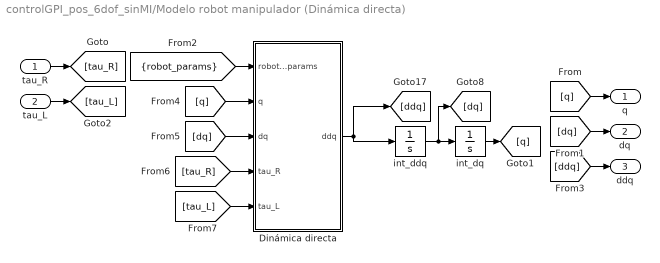
== system controlGPI_pos_6dof_sinMI/Modelo robot manipulador (Dinámica directa) ==
  tau_R : Inport
  tau_L : Inport  Port=2
  Dinámica directa : MATLAB Function  TreatAsAtomicUnit=on
  int_ddq : Integrator  InitialCondition=q_cero
  int_dq : Integrator  InitialCondition=q_eq
  q : Outport
  dq : Outport  Port=2
  ddq : Outport  Port=3
  wires:
  [tau_L] -> Dinámica directa/5(tau_L)
  int_ddq/1 -> [dq], int_dq/1
  [robot_params] -> Dinámica directa/1(robot_params)
  [dq] -> Dinámica directa/3(dq)
  int_dq/1 -> [q]
  [tau_R] -> Dinámica directa/4(tau_R)
  Dinámica directa/1(ddq) -> int_ddq/1, [ddq]
  [q] -> q/1
  [dq] -> dq/1
  [ddq] -> ddq/1
  tau_R/1 -> [tau_R]
  tau_L/1 -> [tau_L]
  [q] -> Dinámica directa/2(q)

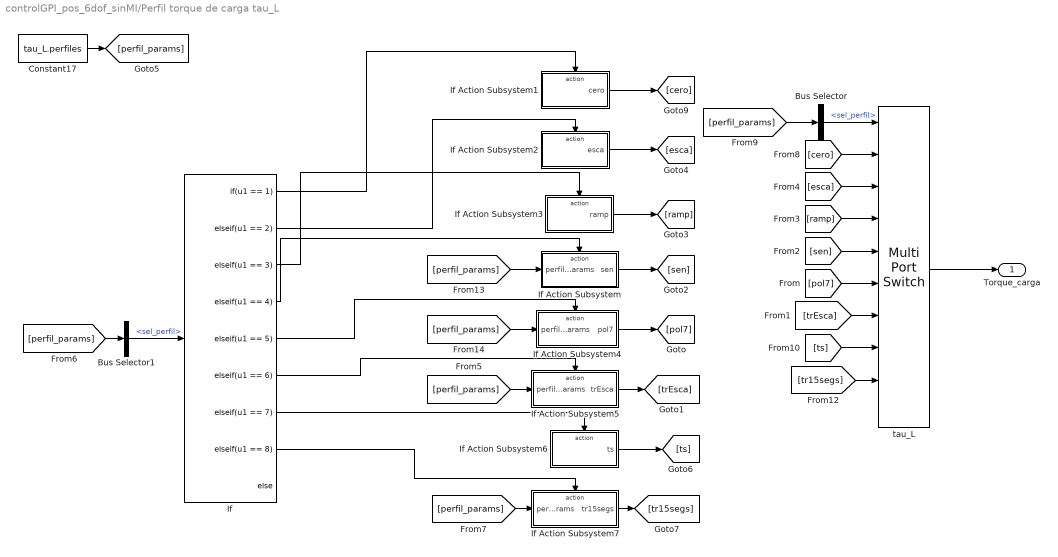
== system controlGPI_pos_6dof_sinMI/Perfil torque de carga tau_L ==
  Bus Selector : BusSelector  OutputSignals=sel_perfil
  Bus Selector1 : BusSelector  OutputSignals=sel_perfil
  Constant17 : Constant  Value=tau_L.perfiles  OutDataTypeStr=Bus: Perfil_bus
  If : If  IfExpression=u1 == 1  ElseIfExpressions=u1 == 2,u1 == 3,u1 == 4,u1 == 5,u1 == 6,u1 == 7,u1 == 8
  If Action Subsystem : Subsystem  TreatAsAtomicUnit=on
  If Action Subsystem1 : Subsystem  TreatAsAtomicUnit=on
  If Action Subsystem2 : Subsystem  TreatAsAtomicUnit=on
  If Action Subsystem3 : Subsystem  TreatAsAtomicUnit=on
  If Action Subsystem4 : Subsystem  TreatAsAtomicUnit=on
  If Action Subsystem5 : Subsystem  TreatAsAtomicUnit=on
  If Action Subsystem6 : Subsystem  TreatAsAtomicUnit=on
  If Action Subsystem7 : Subsystem  TreatAsAtomicUnit=on
  tau_L : MultiPortSwitch  Inputs=9  SaturateOnIntegerOverflow=off  InputSameDT=off
  Torque_carga : Outport
  wires:
  tau_L/1 -> Torque_carga/1
  [ramp] -> tau_L/4
  [trEsca] -> tau_L/7
  [pol7] -> tau_L/6
  [sen] -> tau_L/5
  [esca] -> tau_L/3
  Constant17/1 -> [perfil_params]
  [ts] -> tau_L/8
  [tr15segs] -> tau_L/9
  Bus Selector/1 -> tau_L/1  "<sel_perfil>"
  [perfil_params] -> Bus Selector/1
  If Action Subsystem/1(sen) -> [sen]
  [perfil_params] -> Bus Selector1/1
  Bus Selector1/1 -> If/1  "<sel_perfil>"
  If/4 -> If Action Subsystem/Action
  If Action Subsystem1/1(cero) -> [cero]
  [cero] -> tau_L/2
  [perfil_params] -> If Action Subsystem/1(perfil_params)
  If/1 -> If Action Subsystem1/Action
  If Action Subsystem2/1(esca) -> [esca]
  If/2 -> If Action Subsystem2/Action
  If Action Subsystem3/1(ramp) -> [ramp]
  If/3 -> If Action Subsystem3/Action
  [perfil_params] -> If Action Subsystem4/1(perfil_params)
  If/5 -> If Action Subsystem4/Action
  If Action Subsystem4/1(pol7) -> [pol7]
  If Action Subsystem5/1(trEsca) -> [trEsca]
  [perfil_params] -> If Action Subsystem5/1(perfil_params)
  If Action Subsystem6/1(ts) -> [ts]
  If/6 -> If Action Subsystem5/Action
  If/7 -> If Action Subsystem6/Action
  If Action Subsystem7/1(tr15segs) -> [tr15segs]
  If/8 -> If Action Subsystem7/Action
  [perfil_params] -> If Action Subsystem7/1(perfil_params)

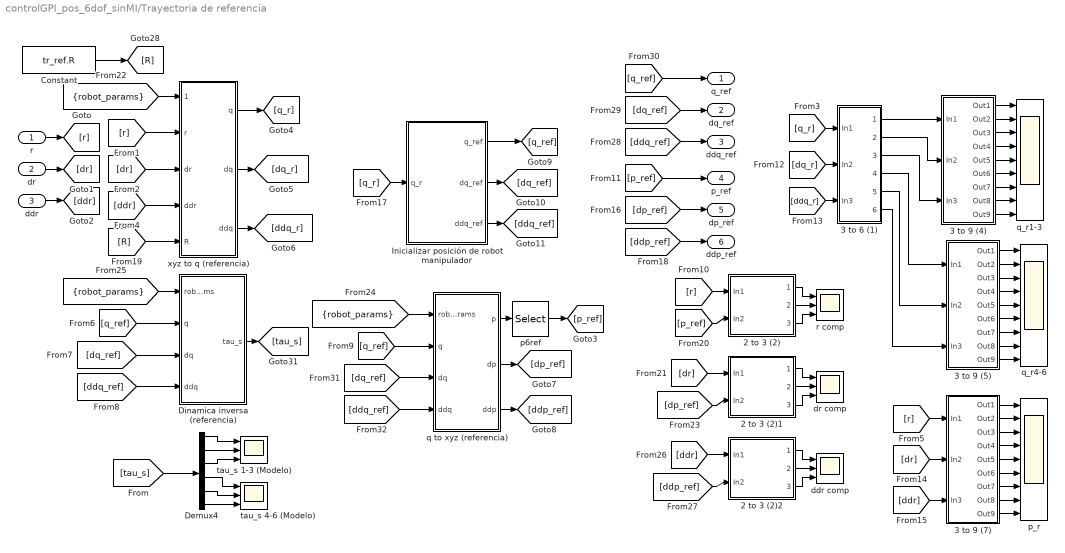
== system controlGPI_pos_6dof_sinMI/Trayectoria de referencia ==
  r : Inport
  dr : Inport  Port=2
  ddr : Inport  Port=3
  2 to 3 (2) : Subsystem
  2 to 3 (2)1 : Subsystem
  2 to 3 (2)2 : Subsystem
  3 to 6 (1) : Subsystem
  3 to 9 (4) : Subsystem
  3 to 9 (5) : Subsystem
  3 to 9 (7) : Subsystem
  Constant : Constant  Value=tr_ref.R
  Demux4 : Demux  Outputs=6
  Dinamica inversa (referencia) : MATLAB Function  TreatAsAtomicUnit=on
  Inicializar posición de robot manipulador : Subsystem
  ddr comp : Scope  NumInputPorts=3
  dr comp : Scope  NumInputPorts=3
  p6ref : Selector  NumberOfDimensions=2  InputPortWidth=3  IndexOptions=Index vector (dialog),Index vector (dialog)  Indices=[1:3],6  OutputSizes=1,1
  p_r : Scope  NumInputPorts=9
  q to xyz (referencia) : MATLAB Function  TreatAsAtomicUnit=on
  q_r1-3 : Scope  NumInputPorts=9
  q_r4-6 : Scope  NumInputPorts=9
  r comp : Scope  NumInputPorts=3
  tau_s 1-3 (Modelo) : Scope  NumInputPorts=3
  tau_s 4-6 (Modelo) : Scope  NumInputPorts=3
  xyz to q (referencia) : MATLAB Function  TreatAsAtomicUnit=on
  q_ref : Outport
  dq_ref : Outport  Port=2
  ddq_ref : Outport  Port=3
  p_ref : Outport  Port=4
  dp_ref : Outport  Port=5
  ddp_ref : Outport  Port=6
  wires:
  xyz to q (referencia)/1(q) -> [q_r]
  [robot_params] -> xyz to q (referencia)/1(robot_params)
  [dq_ref] -> Dinamica inversa (referencia)/3(dq)
  [q_ref] -> Dinamica inversa (referencia)/2(q)
  [q_ref] -> q to xyz (referencia)/2(q)
  [r] -> xyz to q (referencia)/2(r)
  xyz to q (referencia)/2(dq) -> [dq_r]
  q to xyz (referencia)/1(p) -> p6ref/1
  [robot_params] -> Dinamica inversa (referencia)/1(robot_params)
  Dinamica inversa (referencia)/1(tau_s) -> [tau_s]
  xyz to q (referencia)/3(ddq) -> [ddq_r]
  [ddq_ref] -> Dinamica inversa (referencia)/4(ddq)
  [ddr] -> xyz to q (referencia)/4(ddr)
  [dr] -> xyz to q (referencia)/3(dr)
  r/1 -> [r]
  dr/1 -> [dr]
  ddr/1 -> [ddr]
  [tau_s] -> Demux4/1
  [ddq_r] -> 3 to 6 (1)/3(In3)
  [r] -> 3 to 9 (7)/1(In1)
  3 to 9 (7)/7(Out7) -> p_r/7
  [dr] -> 3 to 9 (7)/2(In2)
  3 to 9 (7)/6(Out6) -> p_r/6
  3 to 9 (7)/2(Out2) -> p_r/2
  3 to 9 (7)/9(Out9) -> p_r/9
  [q_r] -> 3 to 6 (1)/1(In1)
  3 to 9 (7)/3(Out3) -> p_r/3
  3 to 9 (7)/1(Out1) -> p_r/1
  3 to 9 (7)/8(Out8) -> p_r/8
  3 to 9 (7)/5(Out5) -> p_r/5
  [dq_r] -> 3 to 6 (1)/2(In2)
  3 to 9 (7)/4(Out4) -> p_r/4
  [ddr] -> 3 to 9 (7)/3(In3)
  [q_r] -> Inicializar posición de robot manipulador/1(q_r)
  3 to 9 (4)/9(Out9) -> q_r1-3/9
  3 to 6 (1)/1(Out1) -> 3 to 9 (4)/1(In1)
  3 to 9 (4)/7(Out7) -> q_r1-3/7
  3 to 9 (5)/2(Out2) -> q_r4-6/2
  3 to 9 (4)/2(Out2) -> q_r1-3/2
  3 to 9 (5)/7(Out7) -> q_r4-6/7
  3 to 9 (5)/9(Out9) -> q_r4-6/9
  3 to 6 (1)/3(Out3) -> 3 to 9 (4)/3(In3)
  3 to 6 (1)/2(Out2) -> 3 to 9 (4)/2(In2)
  3 to 9 (5)/5(Out5) -> q_r4-6/5
  3 to 6 (1)/4(Out4) -> 3 to 9 (5)/1(In1)
  3 to 6 (1)/6(Out6) -> 3 to 9 (5)/3(In3)
  3 to 9 (4)/5(Out5) -> q_r1-3/5
  3 to 9 (4)/6(Out6) -> q_r1-3/6
  3 to 9 (5)/3(Out3) -> q_r4-6/3
  3 to 9 (4)/4(Out4) -> q_r1-3/4
  3 to 9 (5)/1(Out1) -> q_r4-6/1
  3 to 9 (4)/1(Out1) -> q_r1-3/1
  3 to 9 (4)/3(Out3) -> q_r1-3/3
  3 to 9 (5)/6(Out6) -> q_r4-6/6
  3 to 9 (5)/8(Out8) -> q_r4-6/8
  3 to 9 (5)/4(Out4) -> q_r4-6/4
  3 to 6 (1)/5(Out5) -> 3 to 9 (5)/2(In2)
  3 to 9 (4)/8(Out8) -> q_r1-3/8
  Demux4/1 -> tau_s 1-3 (Modelo)/1
  Demux4/6 -> tau_s 4-6 (Modelo)/3
  Demux4/5 -> tau_s 4-6 (Modelo)/2
  Demux4/3 -> tau_s 1-3 (Modelo)/3
  Demux4/4 -> tau_s 4-6 (Modelo)/1
  Demux4/2 -> tau_s 1-3 (Modelo)/2
  Constant/1 -> [R]
  [R] -> xyz to q (referencia)/5(R)
  [robot_params] -> q to xyz (referencia)/1(robot_params)
  2 to 3 (2)/2(2) -> r comp/2
  2 to 3 (2)/1(1) -> r comp/1
  [r] -> 2 to 3 (2)/1(In1)
  2 to 3 (2)/3(3) -> r comp/3
  [p_ref] -> p_ref/1
  [dp_ref] -> dp_ref/1
  [ddp_ref] -> ddp_ref/1
  [p_ref] -> 2 to 3 (2)/2(In2)
  [dp_ref] -> 2 to 3 (2)1/2(In2)
  2 to 3 (2)1/2(2) -> dr comp/2
  2 to 3 (2)1/1(1) -> dr comp/1
  [dr] -> 2 to 3 (2)1/1(In1)
  2 to 3 (2)1/3(3) -> dr comp/3
  [ddp_ref] -> 2 to 3 (2)2/2(In2)
  2 to 3 (2)2/2(2) -> ddr comp/2
  2 to 3 (2)2/1(1) -> ddr comp/1
  [ddr] -> 2 to 3 (2)2/1(In1)
  2 to 3 (2)2/3(3) -> ddr comp/3
  Inicializar posición de robot manipulador/1(q_ref) -> [q_ref]
  Inicializar posición de robot manipulador/2(dq_ref) -> [dq_ref]
  Inicializar posición de robot manipulador/3(ddq_ref) -> [ddq_ref]
  [ddq_ref] -> ddq_ref/1
  [dq_ref] -> dq_ref/1
  [q_ref] -> q_ref/1
  p6ref/1 -> [p_ref]
  [dq_ref] -> q to xyz (referencia)/3(dq)
  [ddq_ref] -> q to xyz (referencia)/4(ddq)
  q to xyz (referencia)/2(dp) -> [dp_ref]
  q to xyz (referencia)/3(ddp) -> [ddp_ref]

== system controlGPI_pos_6dof_sinMI/q to xyz (robot) ==
  q : Inport
  dq : Inport  Port=2
  ddq : Inport  Port=3
  Data Store Memory : DataStoreMemory  DataStoreName=q  WriteAfterWriteMsg=warning  InitialValue=q_eq  ShowAdditionalParam=off
  Data Store Memory1 : DataStoreMemory  DataStoreName=dq  WriteAfterWriteMsg=warning  InitialValue=zeros(size(dq(:,1)))  ShowAdditionalParam=off
  Data Store Memory2 : DataStoreMemory  DataStoreName=ddq  WriteAfterWriteMsg=warning  InitialValue=zeros(size(ddq(:,1)))  ShowAdditionalParam=off
  Data Store Read : DataStoreRead  DataStoreName=q  IndexOptions=Index vector (dialog)  Indices=1  OutputSizes=1
  Data Store Read1 : DataStoreRead  DataStoreName=dq  IndexOptions=Index vector (dialog)  Indices=1  OutputSizes=1
  Data Store Read2 : DataStoreRead  DataStoreName=ddq  IndexOptions=Index vector (dialog)  Indices=1  OutputSizes=1
  Data Store Write : DataStoreWrite  DataStoreName=q  IndexOptions=Index vector (dialog)  Indices=1  OutputSizes=1
  Data Store Write1 : DataStoreWrite  DataStoreName=dq  IndexOptions=Index vector (dialog)  Indices=1  OutputSizes=1
  Data Store Write2 : DataStoreWrite  DataStoreName=ddq  IndexOptions=Index vector (dialog)  Indices=1  OutputSizes=1
  q to xyz (robot) : MATLAB Function  TreatAsAtomicUnit=on
  p : Outport
  dp : Outport  Port=2
  ddp : Outport  Port=3
  wires:
  q/1 -> Data Store Write/1
  dq/1 -> Data Store Write1/1
  ddq/1 -> Data Store Write2/1
  q to xyz (robot)/1(p) -> p/1
  q to xyz (robot)/2(dp) -> dp/1
  q to xyz (robot)/3(ddp) -> ddp/1
  [robot_params] -> q to xyz (robot)/1(robot_params)
  Data Store Read/1 -> q to xyz (robot)/2(q)
  Data Store Read1/1 -> q to xyz (robot)/3(dq)
  Data Store Read2/1 -> q to xyz (robot)/4(ddq)

== system controlGPI_pos_6dof_sinMI/ControladorGPI + NN/2 to 3 (1) ==
  In1 : Inport
  In2 : Inport  Port=2
  Demux : Demux  Outputs=6
  Demux1 : Demux  Outputs=6
  Mux{,1..5} (6 alike) : Mux  Inputs=2
  Out1 : Outport
  Out2 : Outport  Port=2
  Out3 : Outport  Port=3
  Out4 : Outport  Port=4
  Out5 : Outport  Port=5
  Out6 : Outport  Port=6
  wires:
  Demux/3 -> Mux2/1
  Mux2/1 -> Out3/1
  Mux1/1 -> Out2/1
  Demux/1 -> Mux/1
  Demux1/1 -> Mux/2
  In1/1 -> Demux/1
  Demux/2 -> Mux1/1
  Demux1/2 -> Mux1/2
  Mux/1 -> Out1/1
  Demux1/3 -> Mux2/2
  In2/1 -> Demux1/1
  Mux3/1 -> Out4/1
  Mux4/1 -> Out5/1
  Mux5/1 -> Out6/1
  Demux/4 -> Mux3/1
  Demux1/4 -> Mux3/2
  Demux/5 -> Mux4/1
  Demux1/5 -> Mux4/2
  Demux/6 -> Mux5/1
  Demux1/6 -> Mux5/2

== system controlGPI_pos_6dof_sinMI/ControladorGPI + NN/3 to 6 (1)1 ==
  In1 : Inport
  In2 : Inport  Port=2
  In3 : Inport  Port=3
  Demux4 : Demux  Outputs=6
  Demux6 : Demux  Outputs=6
  Demux7 : Demux  Outputs=6
  Mux{,1..5} (6 alike) : Mux  Inputs=3
  Out1 : Outport
  Out2 : Outport  Port=2
  Out3 : Outport  Port=3
  Out4 : Outport  Port=4
  Out5 : Outport  Port=5
  Out6 : Outport  Port=6
  wires:
  Demux6/1 -> Mux2/1
  Demux6/3 -> Mux2/3
  Demux4/2 -> Mux/2
  Demux6/6 -> Mux3/3
  Demux6/2 -> Mux2/2
  Demux6/5 -> Mux3/2
  Mux/1 -> Out1/1
  In1/1 -> Demux4/1
  Demux6/4 -> Mux3/1
  Demux4/1 -> Mux/1
  Demux4/6 -> Mux1/3
  Demux4/4 -> Mux1/1
  Demux7/5 -> Mux5/2
  Demux4/3 -> Mux/3
  Demux4/5 -> Mux1/2
  Demux7/3 -> Mux4/3
  Demux7/1 -> Mux4/1
  Demux7/2 -> Mux4/2
  In3/1 -> Demux7/1
  Mux2/1 -> Out2/1
  Demux7/4 -> Mux5/1
  Demux7/6 -> Mux5/3
  In2/1 -> Demux6/1
  Mux5/1 -> Out6/1
  Mux1/1 -> Out4/1
  Mux4/1 -> Out3/1
  Mux3/1 -> Out5/1

== system controlGPI_pos_6dof_sinMI/ControladorGPI + NN/3 to 9 (6) ==
  In1 : Inport
  In2 : Inport  Port=2
  In3 : Inport  Port=3
  Demux2 : Demux  Outputs=3
  Demux3 : Demux  Outputs=3
  Demux4 : Demux  Outputs=3
  Out1 : Outport
  Out2 : Outport  Port=2
  Out3 : Outport  Port=3
  Out4 : Outport  Port=4
  Out5 : Outport  Port=5
  Out6 : Outport  Port=6
  Out7 : Outport  Port=7
  Out8 : Outport  Port=8
  Out9 : Outport  Port=9
  wires:
  In3/1 -> Demux4/1
  Demux4/1 -> Out3/1
  Demux2/1 -> Out1/1
  Demux3/3 -> Out8/1
  Demux3/2 -> Out5/1
  Demux3/1 -> Out2/1
  In1/1 -> Demux2/1
  Demux2/3 -> Out7/1
  Demux4/3 -> Out9/1
  Demux4/2 -> Out6/1
  Demux2/2 -> Out4/1
  In2/1 -> Demux3/1

== system controlGPI_pos_6dof_sinMI/ControladorGPI + NN/3 to 9 (7) ==
  In1 : Inport
  In2 : Inport  Port=2
  In3 : Inport  Port=3
  Demux2 : Demux  Outputs=3
  Demux3 : Demux  Outputs=3
  Demux4 : Demux  Outputs=3
  Out1 : Outport
  Out2 : Outport  Port=2
  Out3 : Outport  Port=3
  Out4 : Outport  Port=4
  Out5 : Outport  Port=5
  Out6 : Outport  Port=6
  Out7 : Outport  Port=7
  Out8 : Outport  Port=8
  Out9 : Outport  Port=9
  wires:
  In3/1 -> Demux4/1
  Demux4/1 -> Out3/1
  Demux2/1 -> Out1/1
  Demux3/3 -> Out8/1
  Demux3/2 -> Out5/1
  Demux3/1 -> Out2/1
  In1/1 -> Demux2/1
  Demux2/3 -> Out7/1
  Demux4/3 -> Out9/1
  Demux4/2 -> Out6/1
  Demux2/2 -> Out4/1
  In2/1 -> Demux3/1

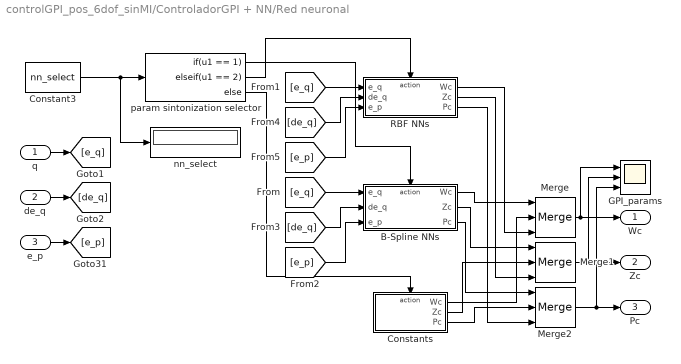
== system controlGPI_pos_6dof_sinMI/ControladorGPI + NN/Red neuronal ==
  q : Inport
  de_q : Inport  Port=2
  e_p : Inport  Port=3
  B-Spline NNs : Subsystem  TreatAsAtomicUnit=on
  Constant3 : Constant  Value=nn_select
  Constants : Subsystem  TreatAsAtomicUnit=on
  GPI_params : Scope  NumInputPorts=3
  Merge : Merge  Inputs=3
  Merge1 : Merge  Inputs=3
  Merge2 : Merge  Inputs=3
  RBF NNs : Subsystem  TreatAsAtomicUnit=on
  nn_select : Display
  param sintonization selector : If  IfExpression=u1 == 1  ElseIfExpressions=u1 == 2
  Wc : Outport
  Zc : Outport  Port=2
  Pc : Outport  Port=3
  wires:
  param sintonization selector/1 -> B-Spline NNs/Action
  B-Spline NNs/1(Wc) -> Merge/1
  param sintonization selector/3 -> Constants/Action
  Constant3/1 -> nn_select/1, param sintonization selector/1
  B-Spline NNs/2(Zc) -> Merge1/1
  B-Spline NNs/3(Pc) -> Merge2/1
  Constants/1(Wc) -> Merge/2
  Constants/2(Zc) -> Merge1/2
  Constants/3(Pc) -> Merge2/2
  q/1 -> [e_q]
  de_q/1 -> [de_q]
  param sintonization selector/2 -> RBF NNs/Action
  RBF NNs/2(Zc) -> Merge1/3
  RBF NNs/1(Wc) -> Merge/3
  RBF NNs/3(Pc) -> Merge2/3
  Merge/1 -> GPI_params/1, Wc/1
  Merge1/1 -> GPI_params/2, Zc/1
  Merge2/1 -> GPI_params/3, Pc/1
  [e_q] -> B-Spline NNs/1(e_q)
  [de_q] -> B-Spline NNs/2(de_q)
  [e_q] -> RBF NNs/1(e_q)
  [de_q] -> RBF NNs/2(de_q)
  e_p/1 -> [e_p]
  [e_p] -> RBF NNs/3(e_p)
  [e_p] -> B-Spline NNs/3(e_p)

== system controlGPI_pos_6dof_sinMI/Perfil torque de carga tau_L/If Action Subsystem ==
  perfil_params : Inport
  Action Port : ActionPort  ActionPortLabel=elseif(u1 == 4)
  Clock2 : Clock
  Clock4 : Clock
  Polinomio 7mo orden sen : MATLAB Function  TreatAsAtomicUnit=on
  Scope1 : Scope
  Scope4 : Scope
  Scope5 : Scope  NumInputPorts=4
  Senoidal tiempo de inicio : MATLAB Function  TreatAsAtomicUnit=on
  Sum1 : Sum  Inputs=|-+
  senoidal : Sin  TimeSource=Use external signal  Frequency=6.2832  Phase=1.5708  SampleTime=0
  sen : Outport
  wires:
  Clock4/1 -> Polinomio 7mo orden sen/1(t)
  Polinomio 7mo orden sen/1(qpol) -> Scope1/1, Sum1/1, Scope5/1
  Sum1/1 -> Scope4/1, [sen]
  Polinomio 7mo orden sen/4(jpol) -> Scope5/4
  Polinomio 7mo orden sen/3(apol) -> Scope5/3
  Clock2/1 -> Senoidal tiempo de inicio/1(t)
  [perfil_params] -> Polinomio 7mo orden sen/2(perfil_params)
  Polinomio 7mo orden sen/2(vpol) -> Scope5/2
  senoidal/1 -> Sum1/2
  Senoidal tiempo de inicio/1(tr) -> senoidal/1
  [sen] -> sen/1
  perfil_params/1 -> [perfil_params]
  [perfil_params] -> Senoidal tiempo de inicio/2(perfil_params)

== system controlGPI_pos_6dof_sinMI/Perfil torque de carga tau_L/If Action Subsystem1 ==
  Action Port : ActionPort  ActionPortLabel=if(u1 == 1)
  Constant : Constant  Value=0
  cero : Outport
  wires:
  Constant/1 -> cero/1

== system controlGPI_pos_6dof_sinMI/Perfil torque de carga tau_L/If Action Subsystem2 ==
  Action Port : ActionPort  ActionPortLabel=elseif(u1 == 2)
  Scope3 : Scope
  Sum : Sum  Inputs=|++
  escalon1 : Step  Time=2.5  After=0.70582  SampleTime=0
  escalon2 : Step  Time=7.5  After=-0.70582  SampleTime=0
  esca : Outport
  wires:
  escalon2/1 -> Sum/2
  escalon1/1 -> Sum/1
  Sum/1 -> [esca], Scope3/1
  [esca] -> esca/1

== system controlGPI_pos_6dof_sinMI/Perfil torque de carga tau_L/If Action Subsystem3 ==
  Action Port : ActionPort  ActionPortLabel=elseif(u1 == 3)
  Scope2 : Scope
  Sum2 : Sum  Inputs=|++
  rampa1 : simulink/Sources/Ramp  slope=0.02064  start=2.5  InitialOutput=0
  rampa2 : simulink/Sources/Ramp  slope=-0.02064  start=7.5  InitialOutput=0
  ramp : Outport
  wires:
  rampa2/1 -> Sum2/2
  rampa1/1 -> Sum2/1
  Sum2/1 -> Scope2/1, [ramp]
  [ramp] -> ramp/1

== system controlGPI_pos_6dof_sinMI/Perfil torque de carga tau_L/If Action Subsystem4 ==
  perfil_params : Inport
  Action Port : ActionPort  ActionPortLabel=elseif(u1 == 5)
  Clock1 : Clock
  Polinomio 7mo orden tau_L : MATLAB Function  TreatAsAtomicUnit=on
  Scope : Scope  NumInputPorts=4
  pol7 : Outport
  wires:
  Polinomio 7mo orden tau_L/4(jpol) -> Scope/4
  Polinomio 7mo orden tau_L/1(qpol) -> Scope/1, [pol7]
  Polinomio 7mo orden tau_L/2(vpol) -> Scope/2
  Clock1/1 -> Polinomio 7mo orden tau_L/1(t)
  Polinomio 7mo orden tau_L/3(apol) -> Scope/3
  perfil_params/1 -> Polinomio 7mo orden tau_L/2(perfil_params)
  [pol7] -> pol7/1

== system controlGPI_pos_6dof_sinMI/Perfil torque de carga tau_L/If Action Subsystem5 ==
  perfil_params : Inport
  Action Port : ActionPort  ActionPortLabel=elseif(u1 == 6)
  Clock : Clock
  Scope1 : Scope
  Tren de esca : MATLAB Function  TreatAsAtomicUnit=on
  trEsca : Outport
  wires:
  Tren de esca/1(q) -> Scope1/1, [trEsca]
  Clock/1 -> Tren de esca/1(t)
  perfil_params/1 -> Tren de esca/2(perfil_params)
  [trEsca] -> trEsca/1

== system controlGPI_pos_6dof_sinMI/Perfil torque de carga tau_L/If Action Subsystem6 ==
  Action Port : ActionPort  ActionPortLabel=elseif(u1 == 7)
  Clock3 : Clock
  Polinomio 7mo orden timeseries : MATLAB Function  TreatAsAtomicUnit=on
  Product : Product
  Scope6 : Scope  NumInputPorts=4
  ts_data1 : FromWorkspace  Commented=on  VariableName=tau_L_ts
  ts : Outport
  wires:
  Product/1 -> [ts]
  Clock3/1 -> Polinomio 7mo orden timeseries/1(t)
  ts_data1/1 -> Product/1
  Polinomio 7mo orden timeseries/4(jpol) -> Scope6/4
  Polinomio 7mo orden timeseries/2(vpol) -> Scope6/2
  Polinomio 7mo orden timeseries/3(apol) -> Scope6/3
  Polinomio 7mo orden timeseries/1(qpol) -> Product/2, Scope6/1
  [ts] -> ts/1

== system controlGPI_pos_6dof_sinMI/Perfil torque de carga tau_L/If Action Subsystem7 ==
  perfil_params : Inport
  Action Port : ActionPort  ActionPortLabel=elseif(u1 == 8)
  Clock5 : Clock
  Scope7 : Scope
  Trayectoria 15 segmentos : MATLAB Function  TreatAsAtomicUnit=on
  tr15segs : Outport
  wires:
  Clock5/1 -> Trayectoria 15 segmentos/1(t)
  Trayectoria 15 segmentos/1(q) -> Scope7/1, [tr15segs]
  [tr15segs] -> tr15segs/1
  perfil_params/1 -> Trayectoria 15 segmentos/2(perfil_params)

== system controlGPI_pos_6dof_sinMI/Trayectoria de referencia/2 to 3 (2) ==
  In1 : Inport
  In2 : Inport  Port=2
  Demux3 : Demux  Outputs=3
  Demux4 : Demux  Outputs=3
  Mux10 : Mux  Inputs=2
  Mux8 : Mux  Inputs=2
  Mux9 : Mux  Inputs=2
  1 : Outport
  2 : Outport  Port=2
  3 : Outport  Port=3
  wires:
  Demux4/3 -> Mux10/2
  Demux3/1 -> Mux8/1
  Demux3/2 -> Mux9/1
  Mux9/1 -> 2/1
  Demux4/2 -> Mux9/2
  Demux4/1 -> Mux8/2
  Demux3/3 -> Mux10/1
  Mux8/1 -> 1/1
  Mux10/1 -> 3/1
  In1/1 -> Demux3/1
  In2/1 -> Demux4/1

== system controlGPI_pos_6dof_sinMI/Trayectoria de referencia/2 to 3 (2)1 ==
  In1 : Inport
  In2 : Inport  Port=2
  Demux3 : Demux  Outputs=3
  Demux4 : Demux  Outputs=3
  Mux10 : Mux  Inputs=2
  Mux8 : Mux  Inputs=2
  Mux9 : Mux  Inputs=2
  1 : Outport
  2 : Outport  Port=2
  3 : Outport  Port=3
  wires:
  Demux4/3 -> Mux10/2
  Demux3/1 -> Mux8/1
  Demux3/2 -> Mux9/1
  Mux9/1 -> 2/1
  Demux4/2 -> Mux9/2
  Demux4/1 -> Mux8/2
  Demux3/3 -> Mux10/1
  Mux8/1 -> 1/1
  Mux10/1 -> 3/1
  In1/1 -> Demux3/1
  In2/1 -> Demux4/1

== system controlGPI_pos_6dof_sinMI/Trayectoria de referencia/2 to 3 (2)2 ==
  In1 : Inport
  In2 : Inport  Port=2
  Demux3 : Demux  Outputs=3
  Demux4 : Demux  Outputs=3
  Mux10 : Mux  Inputs=2
  Mux8 : Mux  Inputs=2
  Mux9 : Mux  Inputs=2
  1 : Outport
  2 : Outport  Port=2
  3 : Outport  Port=3
  wires:
  Demux4/3 -> Mux10/2
  Demux3/1 -> Mux8/1
  Demux3/2 -> Mux9/1
  Mux9/1 -> 2/1
  Demux4/2 -> Mux9/2
  Demux4/1 -> Mux8/2
  Demux3/3 -> Mux10/1
  Mux8/1 -> 1/1
  Mux10/1 -> 3/1
  In1/1 -> Demux3/1
  In2/1 -> Demux4/1

== system controlGPI_pos_6dof_sinMI/Trayectoria de referencia/3 to 6 (1) ==
  In1 : Inport
  In2 : Inport  Port=2
  In3 : Inport  Port=3
  Demux4 : Demux  Outputs=6
  Demux6 : Demux  Outputs=6
  Demux7 : Demux  Outputs=6
  Mux{,1..5} (6 alike) : Mux  Inputs=3
  Out1 : Outport
  Out2 : Outport  Port=2
  Out3 : Outport  Port=3
  Out4 : Outport  Port=4
  Out5 : Outport  Port=5
  Out6 : Outport  Port=6
  wires:
  Demux6/1 -> Mux2/1
  Demux6/3 -> Mux2/3
  Demux4/2 -> Mux/2
  Demux6/6 -> Mux3/3
  Demux6/2 -> Mux2/2
  Demux6/5 -> Mux3/2
  Mux/1 -> Out1/1
  In1/1 -> Demux4/1
  Demux6/4 -> Mux3/1
  Demux4/1 -> Mux/1
  Demux4/6 -> Mux1/3
  Demux4/4 -> Mux1/1
  Demux7/5 -> Mux5/2
  Demux4/3 -> Mux/3
  Demux4/5 -> Mux1/2
  Demux7/3 -> Mux4/3
  Demux7/1 -> Mux4/1
  Demux7/2 -> Mux4/2
  In3/1 -> Demux7/1
  Mux2/1 -> Out2/1
  Demux7/4 -> Mux5/1
  Demux7/6 -> Mux5/3
  In2/1 -> Demux6/1
  Mux5/1 -> Out6/1
  Mux1/1 -> Out4/1
  Mux4/1 -> Out3/1
  Mux3/1 -> Out5/1
